simulink model "octocopterDynamicModel"  (R2019b)
settings: Solver=ode1  StartTime=0.0  StopTime=30  FixedStep=dt  RelTol=1e-3  EnableMultiTasking=on
values from neighbouring files (symbols this model uses):
  alpha = 0    [InitVariable.m]
  dt = 0.01    [InitVariable.m]
  err1Enable = 0    [InitVariable.m]
  err2Enable = 0    [InitVariable.m]
  err3Enable = 0    [InitVariable.m]
  err4Enable = 0    [InitVariable.m]
  err5Enable = 0    [InitVariable.m]
  err6Enable = 0    [InitVariable.m]
  err7Enable = 0    [InitVariable.m]
  err8Enable = 0    [InitVariable.m]
  EulerInt_initial = [0;0;0]    [InitVariable.m]
  gravity = 9.81    [InitVariable.m]
  K1 = 0.5    [InitVariable.m]
  Kd_phi = 1.9    [InitVariable.m]
  Kd_phidot = 0.2    [InitVariable.m]
  Kd_psi = 0.8    [InitVariable.m]
  Kd_psidot = 0.1    [InitVariable.m]
  Kd_theta = 0.7    [InitVariable.m]
  Kd_thetadot = 0.1    [InitVariable.m]
  Kd_vz = 4.2    [InitVariable.m]
  Kd_z = 2.2    [InitVariable.m]
  Ki_phi = 0.5    [InitVariable.m]
  Ki_phidot = 0.3    [InitVariable.m]
  Ki_psi = 0.4    [InitVariable.m]
  Ki_psidot = 0.2    [InitVariable.m]
  Ki_theta = 0.4    [InitVariable.m]
  Ki_thetadot = 0.5    [InitVariable.m]
  Ki_vz = 4    [InitVariable.m]
  Ki_z = 60    [InitVariable.m]
  Kp_phi = 0.9    [InitVariable.m]
  Kp_phidot = 0.9    [InitVariable.m]
  Kp_psi = 1.5    [InitVariable.m]
  Kp_psidot = 1.9    [InitVariable.m]
  Kp_theta = 1.6    [InitVariable.m]
  Kp_thetadot = 1.5    [InitVariable.m]
  Kp_vz = 8    [InitVariable.m]
  Kp_z = 22    [InitVariable.m]
  l1 = 0.45    [InitVariable.m]
  l2 = 0.45    [InitVariable.m]
  mass = 10.0    (= 10)    [InitVariable.m]
  moment_of_inertia = diag([1.0, 1.0, 2.0])    [InitVariable.m]
  motorErr1Time = 0    [InitVariable.m]
  motorErr2Time = 0    [InitVariable.m]
  motorErr3Time = 0    [InitVariable.m]
  motorErr4Time = 0    [InitVariable.m]
  motorErr5Time = 0    [InitVariable.m]
  motorErr6Time = 0    [InitVariable.m]
  motorErr7Time = 0    [InitVariable.m]
  motorErr8Time = 0    [InitVariable.m]
  omegaInt_initial = [0;0;0]    [InitVariable.m]
  phiRefFinal = 0    [InitVariable.m]    (also in exampleCase.m = -0.0872664625997)
  phiRefStepTime = 0    [InitVariable.m]    (also in exampleCase.m = 1)
  PosInertialInt_initial = [0;0;0]    [InitVariable.m]    (also in exampleCase.m = [0;0;-10])
  psiRefFinal = 0    [InitVariable.m]    (also in exampleCase.m = 1.0471975512)
  psiRefStepTime = 0    [InitVariable.m]    (also in exampleCase.m = 1)
  rotor_max_rad_per_s = 30    [InitVariable.m]
  rotor_min_rad_per_s = 0    [InitVariable.m]
  rotor_thrust_coeff = 0.05    [InitVariable.m]
  rotor_torque_coeff = 0.005    [InitVariable.m]
  thetaRefFinal = 0    [InitVariable.m]    (also in exampleCase.m = -0.174532925199)
  thetaRefStepTime = 0    [InitVariable.m]    (also in exampleCase.m = 1)
  vbInt_initial = [0;0;0]    [InitVariable.m]
  zRefFinal = 0    [InitVariable.m]    (also in exampleCase.m = -10)
  zRefStepTime = 0    [InitVariable.m]
Description:
  | Copyright (C) 2022 Dogan Yildiz <doganyildiz1990@gmail.com>
  |      This program is free software: you can redistribute it and/or modify
  |      it under the terms of the GNU General Public License as published by
  |      the Free Software Foundation, either version 3 of the License, or
  |      (at your option) any later version.
  | 
  |     This program is distributed in the hope that it will be useful,
  |      but WITHOUT ANY WARRANTY; without even the implied warranty of
  |      MERCHANTABILITY or FITNESS FOR A PARTICULAR PURPOSE.  See the
  |      GNU General Public License for more details.
settings Model: PauseTimes=1  PacingRate=0.010000  Creator=TrueAdmin  LastModifiedBy=TrueAdmin
settings SolverCC: ConcurrentTasks=on

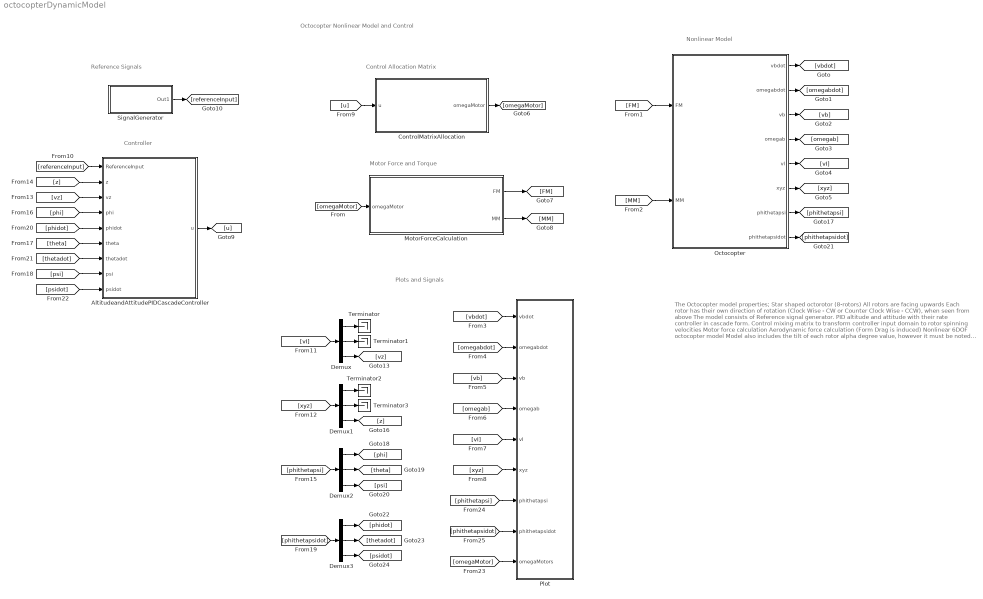
== system octocopterDynamicModel ==
  note: The Octocopter model properties;
      | Star shaped octorotor (8-rotors)
      | All rotors are facing upwards
      | Each rotor has their own direction of rotation
      | (Clock Wise - CW or Counter Clock Wise - CCW), when seen from above
      | The model consists of
      | Reference signal generator.
      | PID altitude and attitude with their rate controller in cascade form.
      | Control mixing matrix to transform controller input domain to rotor spinning velocities
      | Motor force calculation
      | Aerodynamic force calculation (Form Drag is induced)
      | Nonlinear 6DOF octocopter model
      | Model also includes the tilt of each rotor alpha degree value, however it must be noted that
      | this brings extra force ux, uy on octocopter. These values contribution also considered in
      | control mixing calculation.
      |
      | Copyright (C) 2022 Dogan Yildiz <doganyildiz1990@gmail.com>
      | This program is free software: you can redistribute it and/or modify
      | it under the terms of the GNU General Public License as published by
      | the Free Software Foundation, either version 3 of the License, or
      | (at your option) any later version.
      |
      | This program is distributed in the hope that it will be useful,
      | but WITHOUT ANY WARRANTY; without even the implied warranty of
      | MERCHANTABILITY or FITNESS FOR A PARTICULAR PURPOSE. See the
      | GNU General Public License for more details.
      |
      | Department of Electrical - Electronics Engineering
      | Middle East Technical University, METU Teknokent
      | You are free to use this software for academic purposes.
      | For commercial use, please contact the authors.
      | Copyright 2019 The MathWorks, Inc
  note: Controller
  note: Octocopter Nonlinear Model and Control
  note: Nonlinear Model
  note: Control Allocation Matrix
  note: Motor Force and Torque
  note: Plots and Signals
  note: Reference Signals
  AltitudeandAttitudePIDCascadeController : Subsystem
  ControlMatrixAllocation : Subsystem
  Demux{,1..3} (4 alike) : Demux  Outputs=3
  MotorForceCalculation : Subsystem
  Octocopter : Subsystem
  Plot : Subsystem
  SignalGenerator : Subsystem
  Terminator{,1..3} (4 alike) : Terminator
  wires:
  Octocopter/1(vbdot) -> [vbdot]
  Octocopter/2(omegabdot) -> [omegabdot]
  Octocopter/3(vb) -> [vb]
  Octocopter/4(omegab) -> [omegab]
  Octocopter/5(vl) -> [vI]
  Octocopter/6(xyz) -> [xyz]
  ControlMatrixAllocation/1(omegaMotor) -> [omegaMotor]
  [omegaMotor] -> MotorForceCalculation/1(omegaMotor)
  MotorForceCalculation/1(FM) -> [FM]
  MotorForceCalculation/2(MM) -> [MM]
  [FM] -> Octocopter/1(FM)
  [MM] -> Octocopter/2(MM)
  [vbdot] -> Plot/1(vbdot)
  [omegabdot] -> Plot/2(omegabdot)
  [vb] -> Plot/3(vb)
  [omegab] -> Plot/4(omegab)
  [vI] -> Plot/5(vI)
  [xyz] -> Plot/6(xyz)
  AltitudeandAttitudePIDCascadeController/1(u) -> [u]
  SignalGenerator/1(Out1) -> [referenceInput]
  [referenceInput] -> AltitudeandAttitudePIDCascadeController/1(ReferenceInput)
  [vI] -> Demux/1
  Demux/1 -> Terminator/1
  Demux/2 -> Terminator1/1
  Demux/3 -> [vz]
  [xyz] -> Demux1/1
  Demux1/3 -> [z]
  Demux1/2 -> Terminator3/1
  Demux1/1 -> Terminator2/1
  [vz] -> AltitudeandAttitudePIDCascadeController/3(vz)
  [z] -> AltitudeandAttitudePIDCascadeController/2(z)
  Octocopter/7(phithetapsi) -> [phithetapsi]
  Demux2/1 -> [phi]
  Demux2/2 -> [theta]
  Demux2/3 -> [psi]
  [phithetapsi] -> Demux2/1
  [phi] -> AltitudeandAttitudePIDCascadeController/4(phi)
  [psi] -> AltitudeandAttitudePIDCascadeController/8(psi)
  [theta] -> AltitudeandAttitudePIDCascadeController/6(theta)
  Octocopter/8(phithetapsidot) -> [phithetapsidot]
  Demux3/3 -> [psidot]
  Demux3/2 -> [thetadot]
  Demux3/1 -> [phidot]
  [phithetapsidot] -> Demux3/1
  [phidot] -> AltitudeandAttitudePIDCascadeController/5(phidot)
  [thetadot] -> AltitudeandAttitudePIDCascadeController/7(thetadot)
  [psidot] -> AltitudeandAttitudePIDCascadeController/9(psidot)
  [phithetapsi] -> Plot/7(phithetapsi)
  [phithetapsidot] -> Plot/8(phithetapsidot)
  [omegaMotor] -> Plot/9(omegaMotors)
  [u] -> ControlMatrixAllocation/1(u)

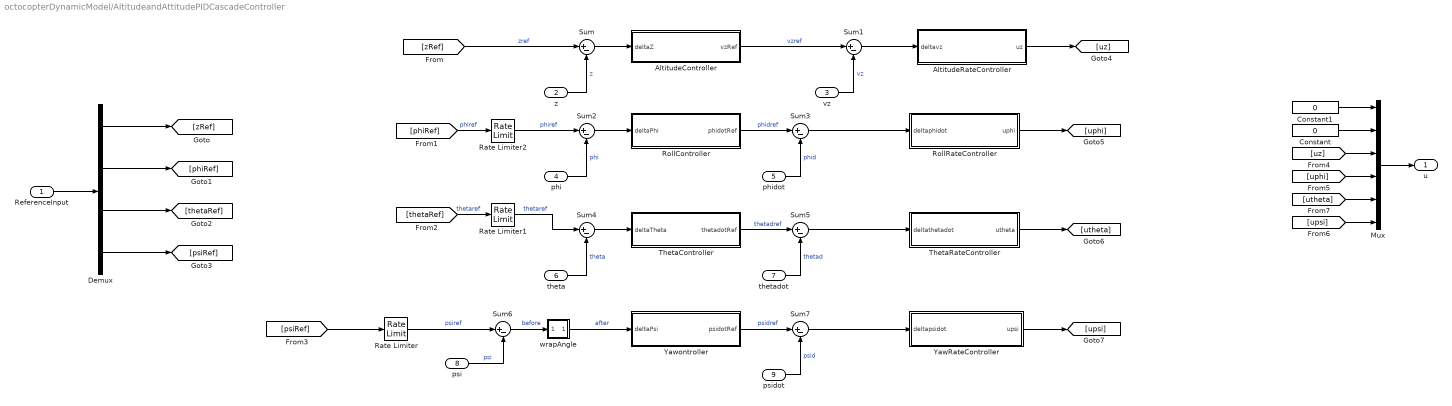
== system octocopterDynamicModel/AltitudeandAttitudePIDCascadeController ==
  ReferenceInput : Inport
  z : Inport  Port=2
  vz : Inport  Port=3
  phi : Inport  Port=4
  phidot : Inport  Port=5
  theta : Inport  Port=6
  thetadot : Inport  Port=7
  psi : Inport  Port=8
  psidot : Inport  Port=9
  AltitudeController : Subsystem
  AltitudeRateController : Subsystem
  Constant : Constant  Value=0
  Constant1 : Constant  Value=0
  Demux : Demux
  Mux : Mux  Inputs=6
  Rate Limiter : RateLimiter  RisingSlewLimit=0.1  FallingSlewLimit=-0.1  SampleTimeMode=inherited
  Rate Limiter1 : RateLimiter  RisingSlewLimit=0.1  FallingSlewLimit=-0.1  SampleTimeMode=inherited
  Rate Limiter2 : RateLimiter  RisingSlewLimit=0.1  FallingSlewLimit=-0.1  SampleTimeMode=inherited
  RollController : Subsystem
  RollRateController : Subsystem
  Sum{,1..7} (8 alike) : Sum  Inputs=|+-
  ThetaController : Subsystem
  ThetaRateController : Subsystem
  YawRateController : Subsystem
  Yawontroller : Subsystem
  wrapAngle : MATLAB Function  TreatAsAtomicUnit=on
  u : Outport
  wires:
  ReferenceInput/1 -> Demux/1
  Demux/1 -> [zRef]
  Demux/2 -> [phiRef]
  Demux/3 -> [thetaRef]
  Demux/4 -> [psiRef]
  [zRef] -> Sum/1  "zref"
  Sum/1 -> AltitudeController/1(deltaZ)
  z/1 -> Sum/2  "z"
  Sum1/1 -> AltitudeRateController/1(deltavz)
  phidot/1 -> Sum3/2  "phid"
  RollController/1(phidotRef) -> Sum3/1  "phidref"
  Sum3/1 -> RollRateController/1(deltaphidot)
  phi/1 -> Sum2/2  "phi"
  Sum2/1 -> RollController/1(deltaPhi)
  Rate Limiter2/1 -> Sum2/1  "phiref"
  Rate Limiter1/1 -> Sum4/1  "thetaref"
  Sum4/1 -> ThetaController/1(deltaTheta)
  theta/1 -> Sum4/2  "theta"
  Sum5/1 -> ThetaRateController/1(deltathetadot)
  ThetaController/1(thetadotRef) -> Sum5/1  "thetadref"
  thetadot/1 -> Sum5/2  "thetad"
  psidot/1 -> Sum7/2  "psid"
  Yawontroller/1(psidotRef) -> Sum7/1  "psidref"
  Sum7/1 -> YawRateController/1(deltapsidot)
  psi/1 -> Sum6/2  "psi"
  Sum6/1 -> wrapAngle/1(u)  "before"
  [psiRef] -> Rate Limiter/1
  AltitudeRateController/1(uz) -> [uz]
  Mux/1 -> u/1
  RollRateController/1(uphi) -> [uphi]
  ThetaRateController/1(utheta) -> [utheta]
  YawRateController/1(upsi) -> [upsi]
  [upsi] -> Mux/6
  [utheta] -> Mux/5
  [uphi] -> Mux/4
  [uz] -> Mux/3
  Constant/1 -> Mux/2
  Constant1/1 -> Mux/1
  vz/1 -> Sum1/2  "vz"
  AltitudeController/1(vzRef) -> Sum1/1  "vzref"
  Rate Limiter/1 -> Sum6/1  "psiref"
  wrapAngle/1(y) -> Yawontroller/1(deltaPsi)  "after"
  [thetaRef] -> Rate Limiter1/1  "thetaref"
  [phiRef] -> Rate Limiter2/1  "phiref"

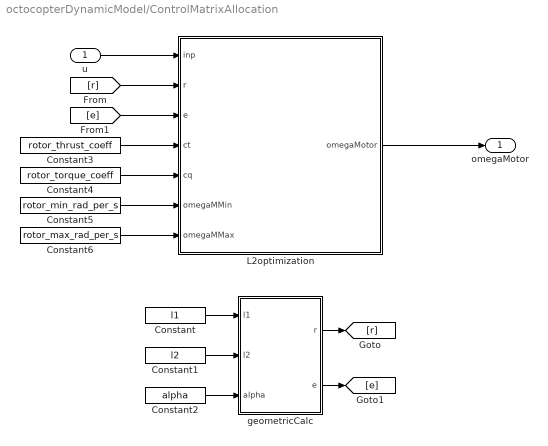
== system octocopterDynamicModel/ControlMatrixAllocation ==
  u : Inport
  Constant : Constant  Value=l1
  Constant1 : Constant  Value=l2
  Constant2 : Constant  Value=alpha
  Constant3 : Constant  Value=rotor_thrust_coeff
  Constant4 : Constant  Value=rotor_torque_coeff
  Constant5 : Constant  Value=rotor_min_rad_per_s
  Constant6 : Constant  Value=rotor_max_rad_per_s
  L2optimization : MATLAB Function  TreatAsAtomicUnit=on  SystemSampleTime=dt
  geometricCalc : MATLAB Function  TreatAsAtomicUnit=on
  omegaMotor : Outport
  wires:
  u/1 -> L2optimization/1(inp)
  Constant2/1 -> geometricCalc/3(alpha)
  Constant1/1 -> geometricCalc/2(l2)
  Constant/1 -> geometricCalc/1(l1)
  geometricCalc/2(e) -> [e]
  geometricCalc/1(r) -> [r]
  [r] -> L2optimization/2(r)
  [e] -> L2optimization/3(e)
  Constant3/1 -> L2optimization/4(ct)
  Constant4/1 -> L2optimization/5(cq)
  Constant5/1 -> L2optimization/6(omegaMMin)
  Constant6/1 -> L2optimization/7(omegaMMax)
  L2optimization/1(omegaMotor) -> omegaMotor/1

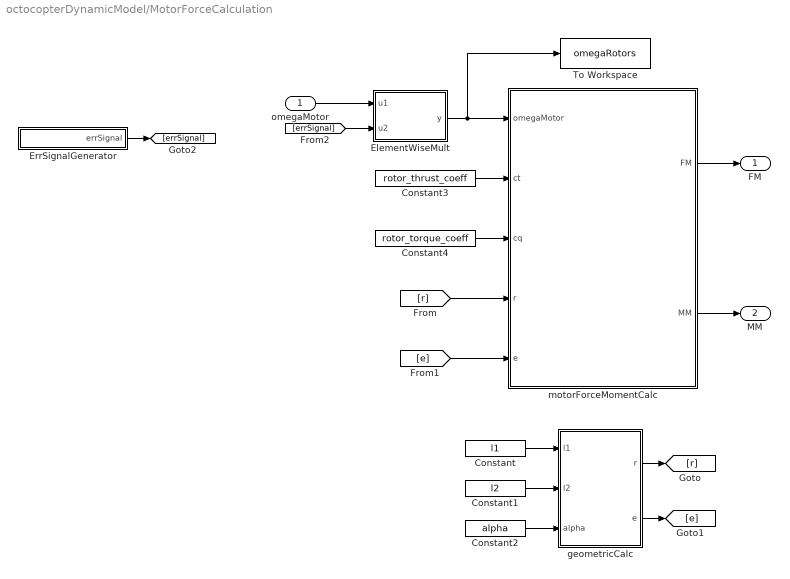
== system octocopterDynamicModel/MotorForceCalculation ==
  omegaMotor : Inport
  Constant : Constant  Value=l1
  Constant1 : Constant  Value=l2
  Constant2 : Constant  Value=alpha
  Constant3 : Constant  Value=rotor_thrust_coeff
  Constant4 : Constant  Value=rotor_torque_coeff
  ElementWiseMult : MATLAB Function  TreatAsAtomicUnit=on  SystemSampleTime=dt
  ErrSignalGenerator : Subsystem
  To Workspace : ToWorkspace  VariableName=omegaRotors  SampleTime=-1
  geometricCalc : MATLAB Function  TreatAsAtomicUnit=on
  motorForceMomentCalc : MATLAB Function  TreatAsAtomicUnit=on
  FM : Outport
  MM : Outport  Port=2
  wires:
  motorForceMomentCalc/1(FM) -> FM/1
  motorForceMomentCalc/2(MM) -> MM/1
  geometricCalc/1(r) -> [r]
  [r] -> motorForceMomentCalc/4(r)
  geometricCalc/2(e) -> [e]
  [e] -> motorForceMomentCalc/5(e)
  Constant/1 -> geometricCalc/1(l1)
  Constant2/1 -> geometricCalc/3(alpha)
  Constant1/1 -> geometricCalc/2(l2)
  Constant3/1 -> motorForceMomentCalc/2(ct)
  Constant4/1 -> motorForceMomentCalc/3(cq)
  omegaMotor/1 -> ElementWiseMult/1(u1)
  ErrSignalGenerator/1(errSignal) -> [errSignal]
  [errSignal] -> ElementWiseMult/2(u2)
  ElementWiseMult/1(y) -> To Workspace/1, motorForceMomentCalc/1(omegaMotor)

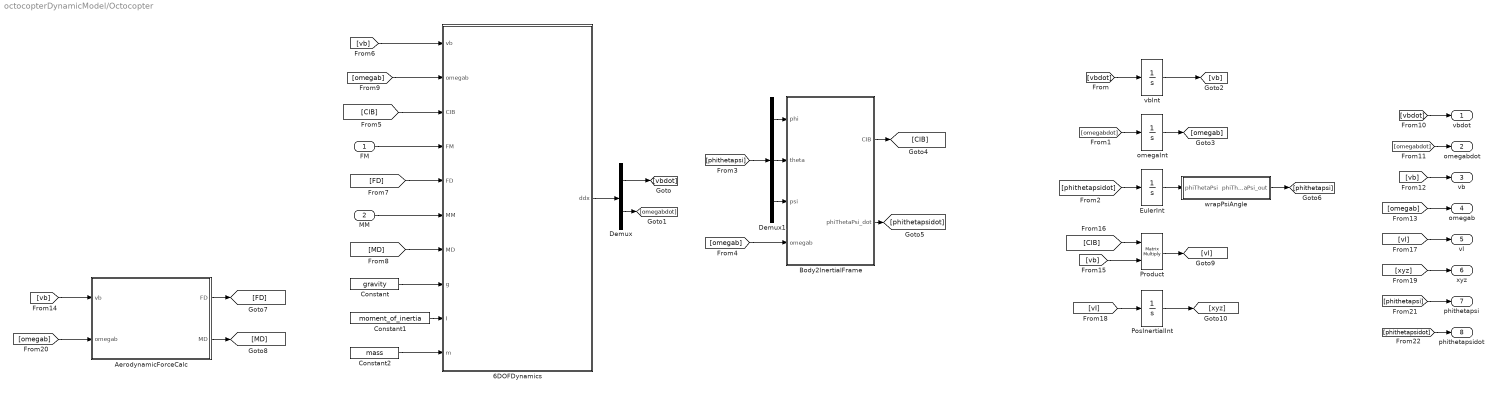
== system octocopterDynamicModel/Octocopter ==
  FM : Inport
  MM : Inport  Port=2
  6DOFDynamics : MATLAB Function  TreatAsAtomicUnit=on
  AerodynamicForceCalc : MATLAB Function  TreatAsAtomicUnit=on
  Body2InertialFrame : MATLAB Function  TreatAsAtomicUnit=on
  Constant : Constant  Value=gravity
  Constant1 : Constant  Value=moment_of_inertia
  Constant2 : Constant  Value=mass
  Demux : Demux  Outputs=[3 3]
  Demux1 : Demux  Outputs=3
  EulerInt : Integrator  InitialCondition=EulerInt_initial
  PosInertialInt : Integrator  InitialCondition=PosInertialInt_initial
  Product : Product  Multiplication=Matrix(*)
  omegaInt : Integrator  InitialCondition=omegaInt_initial  UpperSaturationLimit=rotor_max_rad_per_s  LowerSaturationLimit=rotor_min_rad_per_s
  vbInt : Integrator  InitialCondition=vbInt_initial
  wrapPsiAngle : Subsystem
  vbdot : Outport
  omegabdot : Outport  Port=2
  vb : Outport  Port=3
  omegab : Outport  Port=4
  vl : Outport  Port=5
  xyz : Outport  Port=6
  phithetapsi : Outport  Port=7
  phithetapsidot : Outport  Port=8
  wires:
  6DOFDynamics/1(ddx) -> Demux/1
  Demux/1 -> [vbdot]
  Demux/2 -> [omegabdot]
  [vbdot] -> vbInt/1
  [omegabdot] -> omegaInt/1
  omegaInt/1 -> [omegab]
  vbInt/1 -> [vb]
  Body2InertialFrame/1(CIB) -> [CIB]
  Body2InertialFrame/2(phiThetaPsi_dot) -> [phithetapsidot]
  [phithetapsidot] -> EulerInt/1
  EulerInt/1 -> wrapPsiAngle/1(phiThetaPsi)
  [phithetapsi] -> Demux1/1
  Demux1/1 -> Body2InertialFrame/1(phi)
  Demux1/2 -> Body2InertialFrame/2(theta)
  Demux1/3 -> Body2InertialFrame/3(psi)
  [omegab] -> Body2InertialFrame/4(omegab)
  [CIB] -> 6DOFDynamics/3(CIB)
  [vb] -> 6DOFDynamics/1(vb)
  AerodynamicForceCalc/1(FD) -> [FD]
  AerodynamicForceCalc/2(MD) -> [MD]
  [FD] -> 6DOFDynamics/5(FD)
  [MD] -> 6DOFDynamics/7(MD)
  Constant/1 -> 6DOFDynamics/8(g)
  Constant1/1 -> 6DOFDynamics/9(I)
  Constant2/1 -> 6DOFDynamics/10(m)
  MM/1 -> 6DOFDynamics/6(MM)
  FM/1 -> 6DOFDynamics/4(FM)
  [omegab] -> 6DOFDynamics/2(omegab)
  [vbdot] -> vbdot/1
  [omegabdot] -> omegabdot/1
  [vb] -> vb/1
  [omegab] -> omegab/1
  [vb] -> Product/2
  [CIB] -> Product/1
  Product/1 -> [vI]
  [vI] -> vl/1
  [vI] -> PosInertialInt/1
  PosInertialInt/1 -> [xyz]
  [xyz] -> xyz/1
  wrapPsiAngle/1(phiThetaPsi_out) -> [phithetapsi]
  [vb] -> AerodynamicForceCalc/1(vb)
  [omegab] -> AerodynamicForceCalc/2(omegab)
  [phithetapsi] -> phithetapsi/1
  [phithetapsidot] -> phithetapsidot/1

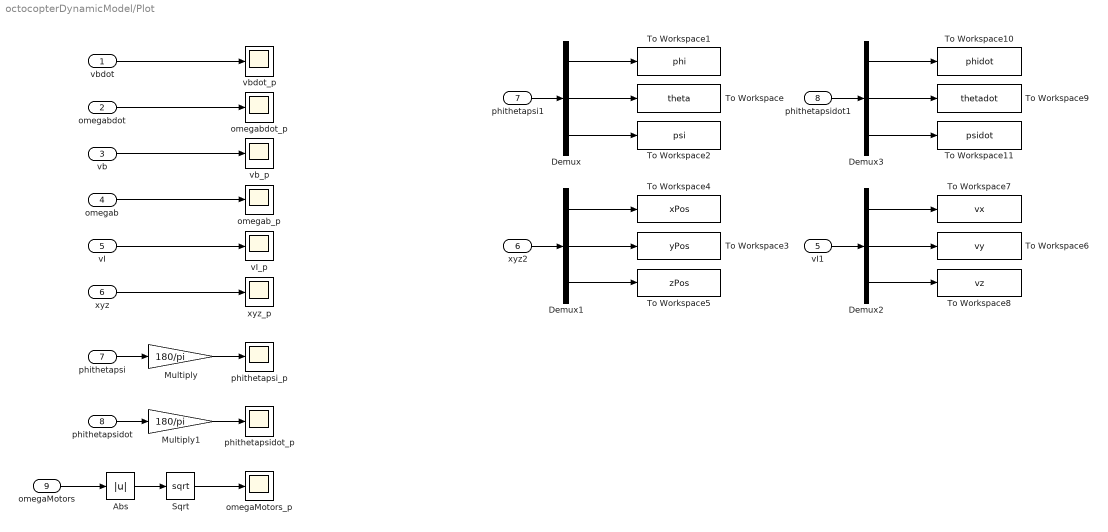
== system octocopterDynamicModel/Plot ==
  vbdot : Inport
  omegabdot : Inport  Port=2
  vb : Inport  Port=3
  omegab : Inport  Port=4
  vI : Inport  Port=5
  xyz : Inport  Port=6
  phithetapsi : Inport  Port=7
  phithetapsidot : Inport  Port=8
  omegaMotors : Inport  Port=9  SampleTime=dt
  Abs : Abs
  Demux{,1..3} (4 alike) : Demux  Outputs=3
  Multiply : Gain  Gain=180/pi
  Multiply1 : Gain  Gain=180/pi
  Sqrt : Sqrt  SaturateOnIntegerOverflow=on
  To Workspace : ToWorkspace  VariableName=theta  SampleTime=-1
  To Workspace1 : ToWorkspace  VariableName=phi  SampleTime=-1
  To Workspace10 : ToWorkspace  VariableName=phidot  SampleTime=-1
  To Workspace11 : ToWorkspace  VariableName=psidot  SampleTime=-1
  To Workspace2 : ToWorkspace  VariableName=psi  SampleTime=-1
  To Workspace3 : ToWorkspace  VariableName=yPos  SampleTime=-1
  To Workspace4 : ToWorkspace  VariableName=xPos  SampleTime=-1
  To Workspace5 : ToWorkspace  VariableName=zPos  SampleTime=-1
  To Workspace6 : ToWorkspace  VariableName=vy  SampleTime=-1
  To Workspace7 : ToWorkspace  VariableName=vx  SampleTime=-1
  To Workspace8 : ToWorkspace  VariableName=vz  SampleTime=-1
  To Workspace9 : ToWorkspace  VariableName=thetadot  SampleTime=-1
  omegaMotors_p : Scope
  omegab_p : Scope
  omegabdot_p : Scope
  phithetapsi1 : InportShadow  Port=7
  phithetapsi_p : Scope
  phithetapsidot1 : InportShadow  Port=8
  phithetapsidot_p : Scope
  vI1 : InportShadow  Port=5
  vI_p : Scope
  vb_p : Scope
  vbdot_p : Scope
  xyz2 : InportShadow  Port=6
  xyz_p : Scope
  wires:
  vbdot/1 -> vbdot_p/1
  omegabdot/1 -> omegabdot_p/1
  vb/1 -> vb_p/1
  omegab/1 -> omegab_p/1
  vI/1 -> vI_p/1
  xyz/1 -> xyz_p/1
  phithetapsi/1 -> Multiply/1
  omegaMotors/1 -> Abs/1
  Abs/1 -> Sqrt/1
  phithetapsidot/1 -> Multiply1/1
  Sqrt/1 -> omegaMotors_p/1
  Multiply/1 -> phithetapsi_p/1
  Multiply1/1 -> phithetapsidot_p/1
  phithetapsi1/1 -> Demux/1
  Demux/2 -> To Workspace/1
  Demux/3 -> To Workspace2/1
  Demux/1 -> To Workspace1/1
  xyz2/1 -> Demux1/1
  Demux1/1 -> To Workspace4/1
  Demux1/3 -> To Workspace5/1
  Demux1/2 -> To Workspace3/1
  vI1/1 -> Demux2/1
  Demux2/1 -> To Workspace7/1
  Demux2/2 -> To Workspace6/1
  Demux2/3 -> To Workspace8/1
  Demux3/3 -> To Workspace11/1
  Demux3/2 -> To Workspace9/1
  Demux3/1 -> To Workspace10/1
  phithetapsidot1/1 -> Demux3/1

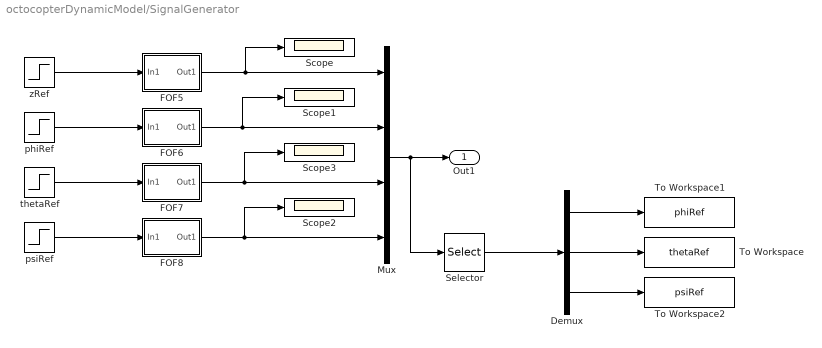
== system octocopterDynamicModel/SignalGenerator ==
  Demux : Demux  Outputs=3
  FOF5 : Subsystem
  FOF6 : Subsystem
  FOF7 : Subsystem
  FOF8 : Subsystem
  Mux : Mux
  Scope{,1..3} (4 alike) : Scope
  Selector : Selector  InputPortWidth=4  IndexOptions=Index vector (dialog)  Indices=[2 3 4]  OutputSizes=1
  To Workspace : ToWorkspace  VariableName=thetaRef  SampleTime=-1
  To Workspace1 : ToWorkspace  VariableName=phiRef  SampleTime=-1
  To Workspace2 : ToWorkspace  VariableName=psiRef  SampleTime=-1
  phiRef : Step  Time=phiRefStepTime  After=phiRefFinal  SampleTime=0
  psiRef : Step  Time=psiRefStepTime  After=psiRefFinal  SampleTime=0
  thetaRef : Step  Time=thetaRefStepTime  After=thetaRefFinal  SampleTime=0
  zRef : Step  Time=zRefStepTime  After=zRefFinal  SampleTime=0
  Out1 : Outport
  wires:
  Mux/1 -> Selector/1, Out1/1
  phiRef/1 -> FOF6/1(In1)
  thetaRef/1 -> FOF7/1(In1)
  psiRef/1 -> FOF8/1(In1)
  zRef/1 -> FOF5/1(In1)
  FOF5/1(Out1) -> Scope/1, Mux/1
  FOF6/1(Out1) -> Scope1/1, Mux/2
  FOF7/1(Out1) -> Scope3/1, Mux/3
  FOF8/1(Out1) -> Scope2/1, Mux/4
  Demux/2 -> To Workspace/1
  Demux/3 -> To Workspace2/1
  Selector/1 -> Demux/1
  Demux/1 -> To Workspace1/1

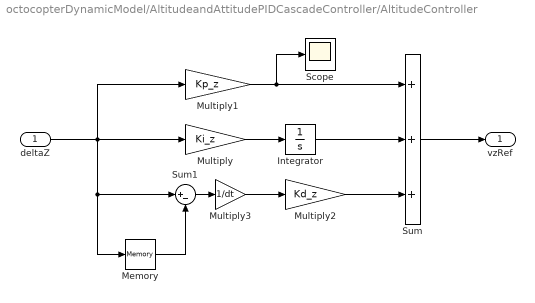
== system octocopterDynamicModel/AltitudeandAttitudePIDCascadeController/AltitudeController ==
  deltaZ : Inport
  Integrator : Integrator
  Memory : Memory
  Multiply : Gain  Gain=Ki_z
  Multiply1 : Gain  Gain=Kp_z
  Multiply2 : Gain  Gain=Kd_z
  Multiply3 : Gain  Gain=1/dt
  Scope : Scope
  Sum : Sum  Inputs=+++
  Sum1 : Sum  Inputs=|+-
  vzRef : Outport
  wires:
  Sum/1 -> vzRef/1
  Multiply/1 -> Integrator/1
  deltaZ/1 -> Multiply/1, Multiply1/1, Sum1/1, Memory/1
  Multiply1/1 -> Scope/1, Sum/1
  Integrator/1 -> Sum/2
  Multiply2/1 -> Sum/3
  Memory/1 -> Sum1/2
  Sum1/1 -> Multiply3/1
  Multiply3/1 -> Multiply2/1

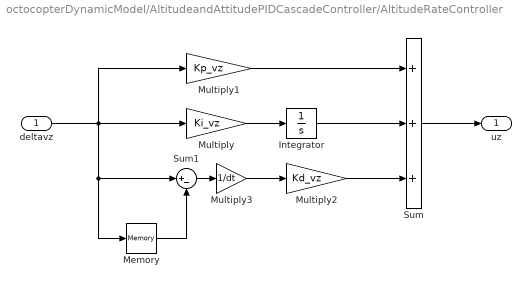
== system octocopterDynamicModel/AltitudeandAttitudePIDCascadeController/AltitudeRateController ==
  deltavz : Inport
  Integrator : Integrator
  Memory : Memory
  Multiply : Gain  Gain=Ki_vz
  Multiply1 : Gain  Gain=Kp_vz
  Multiply2 : Gain  Gain=Kd_vz
  Multiply3 : Gain  Gain=1/dt
  Sum : Sum  Inputs=+++
  Sum1 : Sum  Inputs=|+-
  uz : Outport
  wires:
  Multiply2/1 -> Sum/3
  Multiply3/1 -> Multiply2/1
  Memory/1 -> Sum1/2
  Multiply1/1 -> Sum/1
  Sum/1 -> uz/1
  Multiply/1 -> Integrator/1
  deltavz/1 -> Multiply/1, Multiply1/1, Sum1/1, Memory/1
  Sum1/1 -> Multiply3/1
  Integrator/1 -> Sum/2

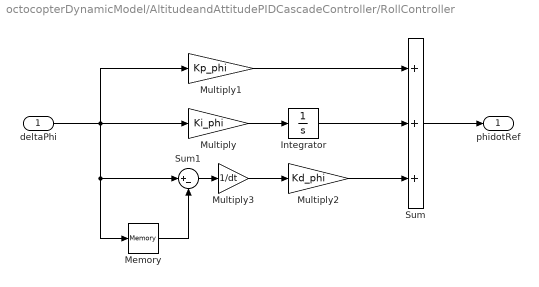
== system octocopterDynamicModel/AltitudeandAttitudePIDCascadeController/RollController ==
  deltaPhi : Inport
  Integrator : Integrator
  Memory : Memory
  Multiply : Gain  Gain=Ki_phi
  Multiply1 : Gain  Gain=Kp_phi
  Multiply2 : Gain  Gain=Kd_phi
  Multiply3 : Gain  Gain=1/dt
  Sum : Sum  Inputs=+++
  Sum1 : Sum  Inputs=|+-
  phidotRef : Outport
  wires:
  Multiply2/1 -> Sum/3
  Multiply3/1 -> Multiply2/1
  Memory/1 -> Sum1/2
  Multiply1/1 -> Sum/1
  Sum/1 -> phidotRef/1
  Multiply/1 -> Integrator/1
  deltaPhi/1 -> Multiply/1, Multiply1/1, Sum1/1, Memory/1
  Sum1/1 -> Multiply3/1
  Integrator/1 -> Sum/2

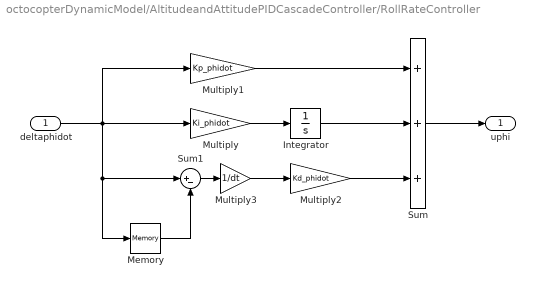
== system octocopterDynamicModel/AltitudeandAttitudePIDCascadeController/RollRateController ==
  deltaphidot : Inport
  Integrator : Integrator
  Memory : Memory
  Multiply : Gain  Gain=Ki_phidot
  Multiply1 : Gain  Gain=Kp_phidot
  Multiply2 : Gain  Gain=Kd_phidot
  Multiply3 : Gain  Gain=1/dt
  Sum : Sum  Inputs=+++
  Sum1 : Sum  Inputs=|+-
  uphi : Outport
  wires:
  Sum/1 -> uphi/1
  Multiply/1 -> Integrator/1
  deltaphidot/1 -> Multiply/1, Multiply1/1, Sum1/1, Memory/1
  Multiply1/1 -> Sum/1
  Memory/1 -> Sum1/2
  Multiply2/1 -> Sum/3
  Multiply3/1 -> Multiply2/1
  Sum1/1 -> Multiply3/1
  Integrator/1 -> Sum/2

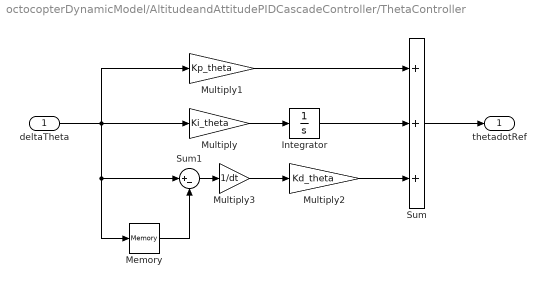
== system octocopterDynamicModel/AltitudeandAttitudePIDCascadeController/ThetaController ==
  deltaTheta : Inport
  Integrator : Integrator
  Memory : Memory
  Multiply : Gain  Gain=Ki_theta
  Multiply1 : Gain  Gain=Kp_theta
  Multiply2 : Gain  Gain=Kd_theta
  Multiply3 : Gain  Gain=1/dt
  Sum : Sum  Inputs=+++
  Sum1 : Sum  Inputs=|+-
  thetadotRef : Outport
  wires:
  deltaTheta/1 -> Multiply/1, Multiply1/1, Sum1/1, Memory/1
  Multiply3/1 -> Multiply2/1
  Multiply2/1 -> Sum/3
  Memory/1 -> Sum1/2
  Sum1/1 -> Multiply3/1
  Integrator/1 -> Sum/2
  Multiply/1 -> Integrator/1
  Multiply1/1 -> Sum/1
  Sum/1 -> thetadotRef/1

== system octocopterDynamicModel/AltitudeandAttitudePIDCascadeController/ThetaRateController ==
  deltathetadot : Inport
  Integrator : Integrator
  Memory : Memory
  Multiply : Gain  Gain=Ki_thetadot
  Multiply1 : Gain  Gain=Kp_thetadot
  Multiply2 : Gain  Gain=Kd_thetadot
  Multiply3 : Gain  Gain=1/dt
  Sum : Sum  Inputs=+++
  Sum1 : Sum  Inputs=|+-
  utheta : Outport
  wires:
  deltathetadot/1 -> Multiply/1, Multiply1/1, Sum1/1, Memory/1
  Multiply3/1 -> Multiply2/1
  Multiply1/1 -> Sum/1
  Sum1/1 -> Multiply3/1
  Integrator/1 -> Sum/2
  Multiply/1 -> Integrator/1
  Multiply2/1 -> Sum/3
  Memory/1 -> Sum1/2
  Sum/1 -> utheta/1

== system octocopterDynamicModel/AltitudeandAttitudePIDCascadeController/YawRateController ==
  deltapsidot : Inport
  Integrator : Integrator
  Memory : Memory
  Multiply : Gain  Gain=Ki_psidot
  Multiply1 : Gain  Gain=Kp_psidot
  Multiply2 : Gain  Gain=Kd_psidot
  Multiply3 : Gain  Gain=1/dt
  Sum : Sum  Inputs=+++
  Sum1 : Sum  Inputs=|+-
  upsi : Outport
  wires:
  deltapsidot/1 -> Multiply/1, Multiply1/1, Sum1/1, Memory/1
  Multiply3/1 -> Multiply2/1
  Multiply1/1 -> Sum/1
  Sum1/1 -> Multiply3/1
  Integrator/1 -> Sum/2
  Multiply/1 -> Integrator/1
  Multiply2/1 -> Sum/3
  Memory/1 -> Sum1/2
  Sum/1 -> upsi/1

== system octocopterDynamicModel/AltitudeandAttitudePIDCascadeController/Yawontroller ==
  deltaPsi : Inport
  Integrator : Integrator
  Memory : Memory
  Multiply : Gain  Gain=Ki_psi
  Multiply1 : Gain  Gain=Kp_psi
  Multiply2 : Gain  Gain=Kd_psi
  Multiply3 : Gain  Gain=1/dt
  Sum : Sum  Inputs=+++
  Sum1 : Sum  Inputs=|+-
  psidotRef : Outport
  wires:
  deltaPsi/1 -> Multiply/1, Multiply1/1, Sum1/1, Memory/1
  Multiply3/1 -> Multiply2/1
  Multiply1/1 -> Sum/1
  Sum1/1 -> Multiply3/1
  Integrator/1 -> Sum/2
  Multiply/1 -> Integrator/1
  Multiply2/1 -> Sum/3
  Memory/1 -> Sum1/2
  Sum/1 -> psidotRef/1

== system octocopterDynamicModel/MotorForceCalculation/ErrSignalGenerator ==
  Mux : Mux  Inputs=8
  motor1 : Subsystem
  motor2 : Subsystem
  motor3 : Subsystem
  motor4 : Subsystem
  motor5 : Subsystem
  motor6 : Subsystem
  motor7 : Subsystem
  motor8 : Subsystem
  errSignal : Outport
  wires:
  Mux/1 -> errSignal/1
  motor1/1(motorErr1Sig) -> Mux/1
  motor2/1(motorErr2Sig) -> Mux/2
  motor3/1(motorErr3Sig) -> Mux/3
  motor4/1(motorErr4Sig) -> Mux/4
  motor5/1(motorErr5Sig) -> Mux/5
  motor6/1(motorErr6Sig) -> Mux/6
  motor7/1(motorErr7Sig) -> Mux/7
  motor8/1(motorErr8Sig) -> Mux/8

== system octocopterDynamicModel/Octocopter/wrapPsiAngle ==
  phiThetaPsi : Inport
  Mux : Mux  Inputs=[2 1]
  Selector : Selector  InputPortWidth=3  IndexOptions=Index vector (dialog)  Indices=[3]  OutputSizes=1
  Selector1 : Selector  InputPortWidth=3  IndexOptions=Index vector (dialog)  Indices=[1 2]  OutputSizes=1
  wrapAngle : MATLAB Function  TreatAsAtomicUnit=on
  phiThetaPsi_out : Outport  VectorParamsAs1DForOutWhenUnconnected=off
  wires:
  Selector/1 -> wrapAngle/1(u)
  phiThetaPsi/1 -> Selector1/1, Selector/1
  wrapAngle/1(y) -> Mux/2
  Mux/1 -> phiThetaPsi_out/1
  Selector1/1 -> Mux/1

== system octocopterDynamicModel/SignalGenerator/FOF5 ==
  In1 : Inport
  Gain : Gain  Gain=K1
  Gain1 : Gain  Gain=K1
  Integrator : Integrator  InitialCondition=PosInertialInt_initial(3,1)
  Sum : Sum  Inputs=|+-
  Out1 : Outport
  wires:
  In1/1 -> Gain/1
  Integrator/1 -> Gain1/1, Out1/1
  Gain/1 -> Sum/1
  Sum/1 -> Integrator/1
  Gain1/1 -> Sum/2

== system octocopterDynamicModel/SignalGenerator/FOF6 ==
  In1 : Inport
  Gain : Gain  Gain=K1
  Gain1 : Gain  Gain=K1
  Integrator : Integrator  InitialCondition=EulerInt_initial(1,1)
  Sum : Sum  Inputs=|+-
  Out1 : Outport
  wires:
  Gain1/1 -> Sum/2
  Sum/1 -> Integrator/1
  Gain/1 -> Sum/1
  Integrator/1 -> Out1/1, Gain1/1
  In1/1 -> Gain/1

== system octocopterDynamicModel/SignalGenerator/FOF7 ==
  In1 : Inport
  Gain : Gain  Gain=K1
  Gain1 : Gain  Gain=K1
  Integrator : Integrator  InitialCondition=EulerInt_initial(2,1)
  Sum : Sum  Inputs=|+-
  Out1 : Outport
  wires:
  In1/1 -> Gain/1
  Integrator/1 -> Gain1/1, Out1/1
  Gain/1 -> Sum/1
  Sum/1 -> Integrator/1
  Gain1/1 -> Sum/2

== system octocopterDynamicModel/SignalGenerator/FOF8 ==
  In1 : Inport
  Gain : Gain  Gain=K1
  Gain1 : Gain  Gain=K1
  Integrator : Integrator  InitialCondition=EulerInt_initial(3,1)
  Sum : Sum  Inputs=|+-
  Out1 : Outport
  wires:
  Gain1/1 -> Sum/2
  Sum/1 -> Integrator/1
  Gain/1 -> Sum/1
  Integrator/1 -> Out1/1, Gain1/1
  In1/1 -> Gain/1

== system octocopterDynamicModel/MotorForceCalculation/ErrSignalGenerator/motor1 ==
  Constant : Constant
  Constant1 : Constant  Value=err1Enable
  Switch : Switch  Criteria=u2 > Threshold
  motorErr1 : Step  Time=motorErr1Time  Before=1  After=0  SampleTime=0
  motorErr1Sig : Outport
  wires:
  Constant1/1 -> Switch/2
  Constant/1 -> Switch/3
  motorErr1/1 -> Switch/1
  Switch/1 -> motorErr1Sig/1

== system octocopterDynamicModel/MotorForceCalculation/ErrSignalGenerator/motor2 ==
  Constant : Constant
  Constant1 : Constant  Value=err2Enable
  Switch : Switch  Criteria=u2 > Threshold
  motorErr2 : Step  Time=motorErr2Time  Before=1  After=0  SampleTime=0
  motorErr2Sig : Outport
  wires:
  Switch/1 -> motorErr2Sig/1
  motorErr2/1 -> Switch/1
  Constant/1 -> Switch/3
  Constant1/1 -> Switch/2

== system octocopterDynamicModel/MotorForceCalculation/ErrSignalGenerator/motor3 ==
  Constant : Constant
  Constant1 : Constant  Value=err3Enable
  Switch : Switch  Criteria=u2 > Threshold
  motorErr3 : Step  Time=motorErr3Time  Before=1  After=0  SampleTime=0
  motorErr3Sig : Outport
  wires:
  Constant1/1 -> Switch/2
  Constant/1 -> Switch/3
  motorErr3/1 -> Switch/1
  Switch/1 -> motorErr3Sig/1

== system octocopterDynamicModel/MotorForceCalculation/ErrSignalGenerator/motor4 ==
  Constant : Constant
  Constant1 : Constant  Value=err4Enable
  Switch : Switch  Criteria=u2 > Threshold
  motorErr4 : Step  Time=motorErr4Time  Before=1  After=0  SampleTime=0
  motorErr4Sig : Outport
  wires:
  Constant1/1 -> Switch/2
  Constant/1 -> Switch/3
  motorErr4/1 -> Switch/1
  Switch/1 -> motorErr4Sig/1

== system octocopterDynamicModel/MotorForceCalculation/ErrSignalGenerator/motor5 ==
  Constant : Constant
  Constant1 : Constant  Value=err5Enable
  Switch : Switch  Criteria=u2 > Threshold
  motorErr5 : Step  Time=motorErr5Time  Before=1  After=0  SampleTime=0
  motorErr5Sig : Outport
  wires:
  Switch/1 -> motorErr5Sig/1
  motorErr5/1 -> Switch/1
  Constant/1 -> Switch/3
  Constant1/1 -> Switch/2

== system octocopterDynamicModel/MotorForceCalculation/ErrSignalGenerator/motor6 ==
  Constant : Constant
  Constant1 : Constant  Value=err6Enable
  Switch : Switch  Criteria=u2 > Threshold
  motorErr6 : Step  Time=motorErr6Time  Before=1  After=0  SampleTime=0
  motorErr6Sig : Outport
  wires:
  Constant1/1 -> Switch/2
  Constant/1 -> Switch/3
  motorErr6/1 -> Switch/1
  Switch/1 -> motorErr6Sig/1

== system octocopterDynamicModel/MotorForceCalculation/ErrSignalGenerator/motor7 ==
  Constant : Constant
  Constant1 : Constant  Value=err7Enable
  Switch : Switch  Criteria=u2 > Threshold
  motorErr7 : Step  Time=motorErr7Time  Before=1  After=0  SampleTime=0
  motorErr7Sig : Outport
  wires:
  Switch/1 -> motorErr7Sig/1
  motorErr7/1 -> Switch/1
  Constant/1 -> Switch/3
  Constant1/1 -> Switch/2

== system octocopterDynamicModel/MotorForceCalculation/ErrSignalGenerator/motor8 ==
  Constant : Constant
  Constant1 : Constant  Value=err8Enable
  Switch : Switch  Criteria=u2 > Threshold
  motorErr8 : Step  Time=motorErr8Time  Before=1  After=0  SampleTime=0
  motorErr8Sig : Outport
  wires:
  Constant1/1 -> Switch/2
  Constant/1 -> Switch/3
  motorErr8/1 -> Switch/1
  Switch/1 -> motorErr8Sig/1

== matlab function octocopterDynamicModel/Octocopter/Body2InertialFrame ==
  data: phi input; CIB output; theta input; psi input; omegab input; phiThetaPsi_dot output
function [CIB,phiThetaPsi_dot] = Body2InertialFrame(phi,theta,psi,omegab)

C3 = [cos(psi) -sin(psi) 0; sin(psi) cos(psi) 0; 0 0 1];
C2 = [cos(theta) 0 sin(theta);0 1 0;-sin(theta) 0 cos(theta)];
C1 = [ 1 0 0; 0 cos(phi) -sin(phi); 0 sin(phi) cos(phi)];

if(mod(theta,pi/2) ~= 0 || theta == 0)
    phiThetaPsi_dot = [1 sin(phi)*tan(theta) cos(phi)*tan(theta);0 cos(phi) -sin(phi); 0 sin(phi)/cos(theta) cos(phi)/cos(theta)]*omegab;
else
    theta = theta + 0.001;
    phiThetaPsi_dot = [1 sin(phi)*tan(theta) cos(phi)*tan(theta);0 cos(phi) -sin(phi); 0 sin(phi)/cos(theta) cos(phi)/cos(theta)]*omegab;    
end

CIB = C3*C2*C1;

== matlab function octocopterDynamicModel/Octocopter/6DOFDynamics ==
  data: vb input; omegab input; CIB input; FM input; FD input; MM input; MD input; g input; I input; m input; ddx output
function ddx  = octoCopter6DOFDynamics(vb,omegab,CIB,FM,FD,MM,MD,g,I,m)

vb_dot     = (1/m)*(FM+FD) + g*CIB'*[0;0;1]-cpmCalc(omegab)*vb;
omegab_dot = I^-1*(MM+MD-cpmCalc(omegab)*(I*omegab));

ddx = [vb_dot;omegab_dot];

end


function cpm_mat = cpmCalc(vec)
    
 cpm_mat = [0          -vec(3,1)   vec(2,1);
            vec(3,1)   0          -vec(1,1);
           -vec(2,1)   vec(1,1)          0];   

end

== matlab function octocopterDynamicModel/Octocopter/AerodynamicForceCalc ==
  data: FD output; MD output; vb input; omegab input
function [FD,MD] = AerodynamicForceCalc(vb,omegab)

rho = 1.2;
CD = 1;
lx=0.2;
ly=0.2;
lz=0.2;
Axy = 0.04;
Axz = 0.04;
Ayz = 0.04;

FD = -0.5*rho*CD*[Ayz*vb(1,1)*abs(vb(1,1));
                  Axz*vb(2,1)*abs(vb(2,1));
                  Axy*vb(3,1)*abs(vb(3,1))];
              
MD = -0.5*rho*CD*[Axy*omegab(1,1)*abs(omegab(1,1))*lx;
                  Axy*omegab(2,1)*abs(omegab(2,1))*ly;
                  8*Ayz*omegab(3,1)*abs(omegab(3,1))*lz];

end

== matlab function octocopterDynamicModel/MotorForceCalculation/motorForceMomentCalc ==
  data: omegaMotor input; FM output; ct input; cq input; MM output; r input; e input
function [FM,MM] = motorForceMomentCalc(omegaMotor,ct,cq,r,e)

TM = ct*omegaMotor;
QM = cq*omegaMotor;

FM = zeros(3,1);

for i = 1:8
    FM  = FM + e(i,:)'*TM(i,1);
end

MM = zeros(3,1);

for i = 1:8
    MM = MM + cpmCalc(r(i,:)')*e(i,:)'*TM(i,1) + (-1)^(i+1)*e(i,:)'*QM(i,1);
end


end


function cpm_mat = cpmCalc(vec)

cpm_mat = [0          -vec(3,1)   vec(2,1);
           vec(3,1)   0          -vec(1,1);
          -vec(2,1)   vec(1,1)          0];

end

== matlab function octocopterDynamicModel/MotorForceCalculation/geometricCalc ==
  data: l1 input; r output; l2 input; alpha input; e output
function [r,e] = geometricCalc(l1,l2,alpha)

k= (1/sqrt(2));

r = [l1   0     0;
     k*l2 k*l2  0;
     0    l1    0;
    -k*l2 k*l2  0;
    -l1   0     0;
    -k*l2 -k*l2 0;
     0    -l1   0;
     k*l2 -k*l2 0];
 
e = [ 0             -sin(alpha)     -cos(alpha);
     -k*sin(alpha)  k*sin(alpha)    -cos(alpha);
      sin(alpha)    0               -cos(alpha);
     -k*sin(alpha)  -k*sin(alpha)   -cos(alpha);
      0             sin(alpha)      -cos(alpha);
      k*sin(alpha)  -k*sin(alpha)   -cos(alpha);
     -sin(alpha)    0               -cos(alpha);
      k*sin(alpha)  k*sin(alpha)    -cos(alpha)];
end

== matlab function octocopterDynamicModel/Octocopter/wrapPsiAngle/wrapAngle ==
  data: u input; y output
function y = wrapAngle(u)
%#codegen
 % Wrap to [0 2*pi]
% y = u - 2*pi*floor(u/(2*pi));
y = u - 2*pi*floor((u+pi)/(2*pi)); % Wrap to [-pi pi]

== matlab function octocopterDynamicModel/ControlMatrixAllocation/L2optimization ==
  data: inp input; omegaMotor output size=8; r input; e input; ct input; cq input; omegaMMin input; omegaMMax input
function omegaMotor = L2optimization(inp,r,e,ct,cq,omegaMMin,omegaMMax)

A = zeros(6,8);
u = zeros(6,1);
coder.varsize('A');
coder.varsize('u');

u = inp;

for j = 1:size(A,2)
    A(1:3,j) = e(j,:)'*ct;
end

for j = 1:size(A,2)
    A(4:6,j) = cpmCalc(r(j,:)')*e(j,:)'*ct+(-1)^(j+1)*e(j,:)'*cq;
end

if(sum(A(1,:)) == 0 && sum(A(2,:)) == 0)
    A =  A(3:6,:);
    u = u(3:6,1);
end

B = [-diag(ones(8,1));diag(ones(8,1))];
c = [-ones(8,1)*omegaMMin^2;ones(8,1)*omegaMMax^2;];

omegaMotor = A'*(A*A')^(-1)*u; 

%KKT Condition check
checkKKT = (B*abs(omegaMotor)<=c)==0;

if(sum(checkKKT==1)~= 0)
    u = priorityAlg(u,A,omegaMMin,omegaMMax);
    omegaMotor = A'*(A*A')^(-1)*u;
end

for i = 1:8
    if(omegaMotor(i,1)>omegaMMax^2)
        omegaMotor(i,1) = omegaMMax^2;
    end
    if(omegaMotor(i,1)<omegaMMin^2)
        omegaMotor(i,1) = omegaMMax^2;
    end
end
end


function cpm_mat = cpmCalc(vec)

cpm_mat = [0          -vec(3,1)   vec(2,1);
           vec(3,1)   0          -vec(1,1);
          -vec(2,1)   vec(1,1)          0];

end

function u= priorityAlg(u,A,omegaMMin,omegaMMax)

if(checkControl(u,A,omegaMMin,omegaMMax))
    return;
end

if (size(u,1) == 6)
    u(1,1) = 0;
    u(2,1) = 0;
    
    if(checkControl(u,A,omegaMMin,omegaMMax))
        return;
    end
    
    h = 0.1;
    n_psi = ceil(abs(u(6,1))/h);
    
    for i = 1:n_psi
        u(6,1) = reduceControl(u(6,1),h);
        if(checkControl(u,A,omegaMMin,omegaMMax))
            return;
        end
    end
    
    u(6,1) = 0;
    
    n_phitheta = ceil(max(abs([u(4,1) u(5,1)]/h)));
    
    for i = 1:n_phitheta
        u(4,1) = reduceControl(u(4,1),h);
        u(5,1) = reduceControl(u(5,1),h);
        if(checkControl(u,A,omegaMMin,omegaMMax))
            return;
        end
    end
    
    u(4,1) = 0;
    u(5,1) = 0;
    
    return;
else
    
    h = 0.1;
    n_psi = ceil(abs(u(4,1))/h);
    
    for i = 1:n_psi
        u(4,1) = reduceControl(u(4,1),h);
        if(checkControl(u,A,omegaMMin,omegaMMax))
            return;
        end
    end
    
    u(4,1) = 0;
    
    n_phitheta = ceil(max(abs([u(2,1) u(3,1)]/h)));
    
    for i = 1:n_phitheta
        u(2,1) = reduceControl(u(2,1),h);
        u(3,1) = reduceControl(u(3,1),h);
        if(checkControl(u,A,omegaMMin,omegaMMax))
            return;
        end
    end
    
    u(2,1) = 0;
    u(3,1) = 0;
    
    return;
    
    
    
end

end

function logicCheck = checkControl(u,A,omegaMMin,omegaMMax)
omegaMotor = A'*(A*A')^(-1)*u; 
logicCheck = 1;
for i = 1:8
    if(sqrt(abs(omegaMotor(i,1)))<omegaMMin || sqrt(abs(omegaMotor(i,1)))>omegaMMax)
        logicCheck = 0;
        break
    end
end
end

function u = reduceControl(u,h)

if(abs(u)>h)
    u = u - sign(u)*h;
else
    u = 0;
end

end

== matlab function octocopterDynamicModel/ControlMatrixAllocation/geometricCalc ==
  data: l1 input; r output; l2 input; alpha input; e output
function [r,e] = geometricCalc(l1,l2,alpha)

k= (1/sqrt(2));

r = [l1   0     0;
     k*l2 k*l2  0;
     0    l1    0;
    -k*l2 k*l2  0;
    -l1   0     0;
    -k*l2 -k*l2 0;
     0    -l1   0;
     k*l2 -k*l2 0];
 
e = [ 0             -sin(alpha)     -cos(alpha);
     -k*sin(alpha)  k*sin(alpha)    -cos(alpha);
      sin(alpha)    0               -cos(alpha);
     -k*sin(alpha)  -k*sin(alpha)   -cos(alpha);
      0             sin(alpha)      -cos(alpha);
      k*sin(alpha)  -k*sin(alpha)   -cos(alpha);
     -sin(alpha)    0               -cos(alpha);
      k*sin(alpha)  k*sin(alpha)    -cos(alpha)];
end

== matlab function octocopterDynamicModel/MotorForceCalculation/ElementWiseMult ==
  data: u1 input; y output; u2 input
function y = fcn(u1,u2)

y = u1.*u2;

== matlab function octocopterDynamicModel/AltitudeandAttitudePIDCascadeController/wrapAngle ==
  data: u input; y output
function y = wrapAngle(u)
%#codegen
 % Wrap to [0 2*pi]
% y = u - 2*pi*floor(u/(2*pi));
y = u - 2*pi*floor((u+pi)/(2*pi)); % Wrap to [-pi pi]
